simulink model "Subsystem"  (R2020a)
settings: Solver=FixedStepAuto  StartTime=0.0  StopTime=10.0  FixedStep=0.2  RelTol=1e-3
model workspace (MAT data in the model file):
  gainA = 2
  gainB = -1
  gainC = 1
  gainD = -1
settings Model: Creator=INDRAJIT MARATHE  LastModifiedBy=INDRAJIT MARATHE
settings DataIOCC: SaveOutput=off  SaveTime=off

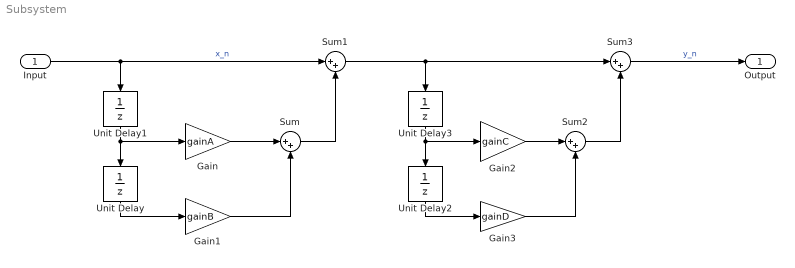
== system Subsystem ==
  Input : Inport  OutDataTypeStr=double  PortDimensions=1  SampleTime=[0.20000000000000001,0]
  Gain : Gain  Gain=gainA
  Gain1 : Gain  Gain=gainB
  Gain2 : Gain  Gain=gainC
  Gain3 : Gain  Gain=gainD
  Sum{,1..3} (4 alike) : Sum  Inputs=|++
  Unit Delay{,1..3} (4 alike) : UnitDelay  SampleTime=-1  HasFrameUpgradeWarning=on
  Output : Outport  OutDataTypeStr=double  PortDimensions=1  SampleTime=[0.20000000000000001,0]
  wires:
  Unit Delay1/1 -> Unit Delay/1, Gain/1
  Sum3/1 -> Output/1  "y_n"
  Sum1/1 -> Unit Delay3/1, Sum3/1
  Input/1 -> Unit Delay1/1, Sum1/1  "x_n"
  Gain1/1 -> Sum/2
  Unit Delay/1 -> Gain1/1
  Gain3/1 -> Sum2/2
  Sum/1 -> Sum1/2
  Gain/1 -> Sum/1
  Sum2/1 -> Sum3/2
  Unit Delay3/1 -> Unit Delay2/1, Gain2/1
  Gain2/1 -> Sum2/1
  Unit Delay2/1 -> Gain3/1
